simulink model "ModelNL1"  (R2018a)
settings: Solver=VariableStepAuto  StartTime=0.0  StopTime=10.0  RelTol=1e-3
values from neighbouring files (symbols this model uses):
  covProcess = 10*diag([0.018^2,(0.018*10)^2,0.018^2,(0.018*10)^2,0.025^2])    [CEEProject.m]    (also in MCsynthesis.m = 1*diag([0.018^2,(0.018*10)^2,0.018^2,(0.018*10)^2,0.025^2]))
  covSensor = (0.018^2)*eye(2)    [CEEProject.m]    (also in MCsynthesis.m)
  D_ = [0 0]    [7_8.m]    (also in CEEProject.m; CEEproject.m; Ines.m; MCsynthesis.m)
  deadzone_u = 5e-2    (= 0.05)    [CEEProject.m]    (also in MCsynthesis.m = 0)
  L = lqe(A, G, C, Qe, Re)    [7_8.m]    (also in CEEProject.m; CEEproject.m; Ines.m; MCsynthesis.m)
  saturation_u = 5    [CEEProject.m]    (also in MCsynthesis.m)
  tc = (1/100)*2*pi/737    (= 8.52535319834e-05)    [CEEProject.m]    (also in MCsynthesis.m)
  V = A - B*K - L*C    [7_8.m]    (also in CEEProject.m; CEEproject.m; Ines.m; MCsynthesis.m)
  x0 = [pi,0,0.1,0,0]'    [7_8.m]    (also in CEEProject.m = [0.1,0,0,0,0]'; CEEproject.m = [0.1,0,0,0,0]'; Ines.m = [pi,0,0.4,0,0]'; MCsynthesis.m = [pi/2,0,0.18,0,0]')
undefined symbols (not defined in the file or in its folder): A, B, C, K
libraries: simulink x4
settings Model: Creator=miguelsilva  LastModifiedBy=leonardopedroso
settings DebuggingCC: LibraryContextMissingDiagnostic=warning
settings SFSimCC: SimUseLocalCustomCode=on
settings RTWCC: RTWUseLocalCustomCode=on

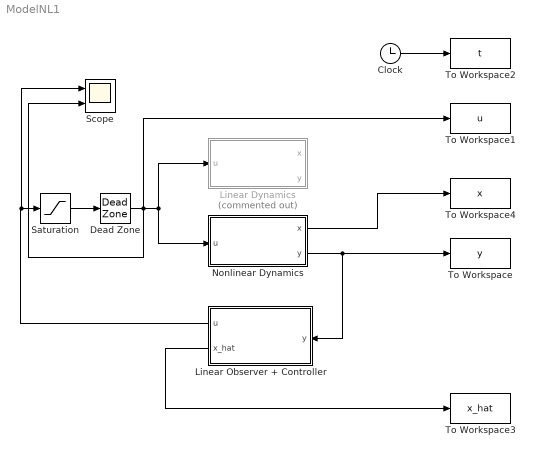
== system ModelNL1 ==
  Clock : Clock
  Dead Zone : DeadZone  LowerValue=-deadzone_u  UpperValue=deadzone_u  SaturateOnIntegerOverflow=on
  Linear Observer + Controller : Subsystem
  Linear Dynamics : Subsystem  Commented=on
  Nonlinear Dynamics : Subsystem
  "Saturation " : Saturate  UpperLimit=saturation_u  LowerLimit=-saturation_u
  Scope : Scope  NumInputPorts=2
  To Workspace : ToWorkspace  VariableName=y  SampleTime=-1
  To Workspace1 : ToWorkspace  VariableName=u  SampleTime=-1
  To Workspace2 : ToWorkspace  VariableName=t  SampleTime=-1
  To Workspace3 : ToWorkspace  VariableName=x_hat  SampleTime=-1
  To Workspace4 : ToWorkspace  VariableName=x  SampleTime=-1
  wires:
  Clock/1 -> To Workspace2/1
  "Saturation "/1 -> Dead Zone/1
  Nonlinear Dynamics/1(x) -> To Workspace4/1
  Nonlinear Dynamics/2(y) -> Linear Observer + Controller/1(y), To Workspace/1
  Linear Observer + Controller/1(u) -> Scope/1, "Saturation "/1
  Linear Observer + Controller/2(x_hat) -> To Workspace3/1
  Dead Zone/1 -> Scope/2, To Workspace1/1, Linear Dynamics/1(u), Nonlinear Dynamics/1(u)

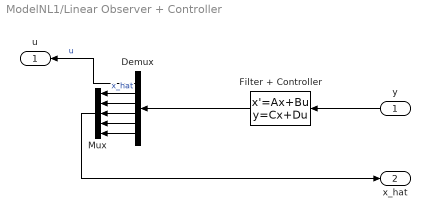
== system ModelNL1/Linear Observer + Controller ==
  y : Inport
  Demux : Demux  Outputs=6
  Filter + Controller : StateSpace  A=V  B=L  C=[-K; eye(5)]  D=[D_;zeros(5,2)]  InitialCondition=0  ContinuousStateAttributes={'y1','y2','y3','y4','y5'}
  Mux : Mux  Inputs=5
  u : Outport
  x_hat : Outport  Port=2
  wires:
  Mux/1 -> x_hat/1
  Demux/1 -> u/1  "u"
  Demux/2 -> Mux/1  "x_hat"
  Demux/5 -> Mux/4
  Demux/3 -> Mux/2
  y/1 -> Filter + Controller/1
  Demux/6 -> Mux/5
  Demux/4 -> Mux/3
  Filter + Controller/1 -> Demux/1

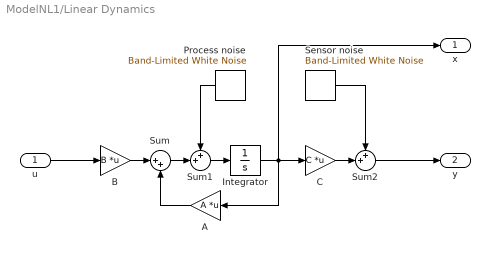
== system ModelNL1/Linear Dynamics ==
  u : Inport
  A : Gain  Gain=A  Multiplication=Matrix(K*u) (u vector)
  B : Gain  Gain=B  Multiplication=Matrix(K*u) (u vector)
  C : Gain  Gain=C  Multiplication=Matrix(K*u) (u vector)
  Integrator : Integrator  InitialCondition=x0
  Process noise : simulink/Sources/Band-Limited White Noise  Cov=diag(covProcess)*tc  Ts=tc  seed=[23341]
  Sensor noise : simulink/Sources/Band-Limited White Noise  Cov=diag(covSensor)*tc  Ts=tc  seed=[23341]
  Sum : Sum  Inputs=|++
  Sum1 : Sum  Inputs=++|
  Sum2 : Sum  Inputs=++|
  x : Outport
  y : Outport  Port=2
  wires:
  u/1 -> B/1
  Sum2/1 -> y/1
  Sum/1 -> Sum1/2
  Process noise/1 -> Sum1/1
  B/1 -> Sum/1
  Sum1/1 -> Integrator/1
  A/1 -> Sum/2
  Integrator/1 -> x/1, C/1, A/1
  Sensor noise/1 -> Sum2/1
  C/1 -> Sum2/2

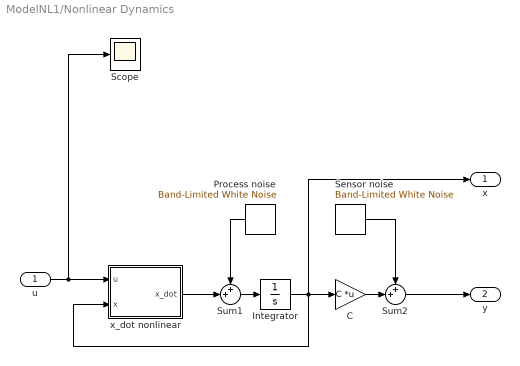
== system ModelNL1/Nonlinear Dynamics ==
  u : Inport
  C : Gain  Gain=C  Multiplication=Matrix(K*u) (u vector)
  Integrator : Integrator  InitialCondition=x0
  Process noise : simulink/Sources/Band-Limited White Noise  Cov=diag(covProcess)*tc  Ts=tc  seed=[23341]
  Scope : Scope
  Sensor noise : simulink/Sources/Band-Limited White Noise  Cov=diag(covSensor)*tc  Ts=tc  seed=[23341]
  Sum1 : Sum  Inputs=++|
  Sum2 : Sum  Inputs=++|
  x_dot nonlinear : MATLAB Function  TreatAsAtomicUnit=on
  x : Outport
  y : Outport  Port=2
  wires:
  Sum2/1 -> y/1
  x_dot nonlinear/1(x_dot) -> Sum1/2
  Process noise/1 -> Sum1/1
  Sum1/1 -> Integrator/1
  Integrator/1 -> x_dot nonlinear/2(x), x/1, C/1
  Sensor noise/1 -> Sum2/1
  C/1 -> Sum2/2
  u/1 -> Scope/1, x_dot nonlinear/1(u)

== matlab function ModelNL1/Nonlinear Dynamics/x_dot nonlinear ==
  data: u input; x_dot output; x input; NLM parameter
function x_dot = x_dot(u,x,NLM)

x_dot = zeros(5,1);
x_dot(1) = x(2);
x_dot(2) = (-NLM.J2*(NLM.Ka1*x(2)-NLM.Kf*x(5)+...
    x(4)*(NLM.Lcm2*NLM.Le1*NLM.m2*x(4)+2*NLM.J2*x(2)*cos(x(3)))*sin(x(3)))+...
    NLM.Lcm2*NLM.Le1*NLM.m2*cos(x(3))*(-NLM.Ka2*x(4)+(NLM.g*NLM.Lcm2*NLM.m2+NLM.J2*x(2)^2*cos(x(3)))*sin(x(3))))/...
    (-NLM.Lcm2^2*NLM.Le1^2*NLM.m2^2*cos(x(3))^2+NLM.J2*(NLM.J0+NLM.J2*sin(x(3))^2));
x_dot(3) = x(4);
x_dot(4) = (NLM.J0*NLM.Ka2*x(4)-NLM.g*NLM.Lcm2*NLM.m2*sin(x(3))*(NLM.J0+NLM.J2*sin(x(3))^2)+...
    cos(x(3))*((-NLM.J0*NLM.J2*x(2)^2+NLM.Lcm2^2*NLM.Le1^2*NLM.m2^2*x(4)^2)*sin(x(3))-...
    NLM.J2^2*x(2)^2*sin(x(3))^3+NLM.Lcm2*NLM.Le1*NLM.m2*(NLM.Ka1*x(2)-NLM.Kf*x(5)+NLM.J2*x(2)*x(4)*sin(2*x(3)))))/...
    (NLM.Lcm2^2*NLM.Le1^2*NLM.m2^2*cos(x(3))^2-NLM.J2*(NLM.J0+NLM.J2*sin(x(3))^2));
x_dot(5) = (-NLM.Kt*x(2)-NLM.R*x(5)+u(1))/NLM.Lb;
